simulink model "PitchRateLimiter"  (R2023b)
settings: Solver=FixedStepDiscrete  StartTime=0.0  StopTime=4  FixedStep=Sample_time  RelTol=1e-3
undefined symbols (not defined in the file): q_fallback_command, q_limit_normal, Sample_time
Description:
  | Illustrative 50 Hz pitch-rate command magnitude limiter. Valid normal-mode inputs are clamped inclusively to plus/minus q_limit_normal; invalid or non-normal inputs use q_fallback_command.
settings Model: DataDictionary=FCS_Data.sldd  Creator=Tyler  LastModifiedBy=Tyler
settings CodeAppCC: MaxIdLength=63

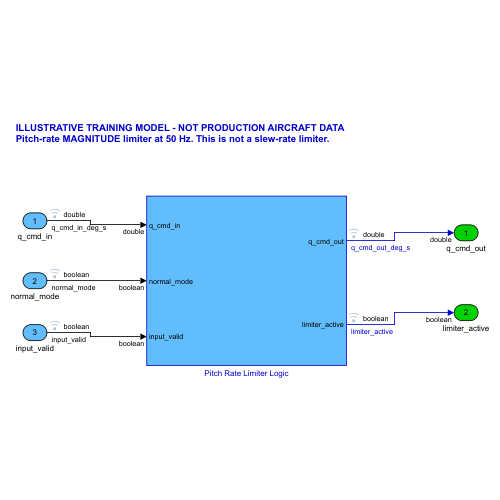
[thumbnail: Simulink's stored preview of the top-level diagram]
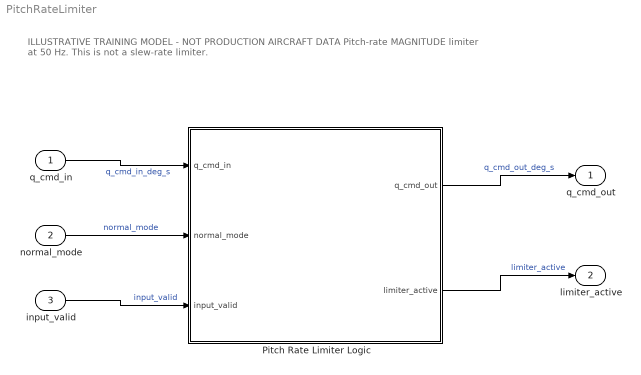
== system PitchRateLimiter ==
  note: ILLUSTRATIVE TRAINING MODEL - NOT PRODUCTION AIRCRAFT DATA
      | Pitch-rate MAGNITUDE limiter at 50 Hz. This is not a slew-rate limiter.
  q_cmd_in : Inport  OutDataTypeStr=double  Unit=deg/s  SampleTime=Sample_time
  normal_mode : Inport  Port=2  OutDataTypeStr=boolean  Unit=1  SampleTime=Sample_time
  input_valid : Inport  Port=3  OutDataTypeStr=boolean  Unit=1  SampleTime=Sample_time
  Pitch Rate Limiter Logic : Subsystem  Description=Inclusive magnitude clamp plus explicit validity/mode fallback. limiter_active is true only while a valid command exceeds a limit.
  q_cmd_out : Outport  OutDataTypeStr=double  Unit=deg/s
  limiter_active : Outport  Port=2  OutDataTypeStr=boolean  Unit=1
  wires:
  q_cmd_in/1 -> Pitch Rate Limiter Logic/1(q_cmd_in)  "q_cmd_in_deg_s"
  normal_mode/1 -> Pitch Rate Limiter Logic/2(normal_mode)  "normal_mode"
  input_valid/1 -> Pitch Rate Limiter Logic/3(input_valid)  "input_valid"
  Pitch Rate Limiter Logic/1(q_cmd_out) -> q_cmd_out/1  "q_cmd_out_deg_s"
  Pitch Rate Limiter Logic/2(limiter_active) -> limiter_active/1  "limiter_active"

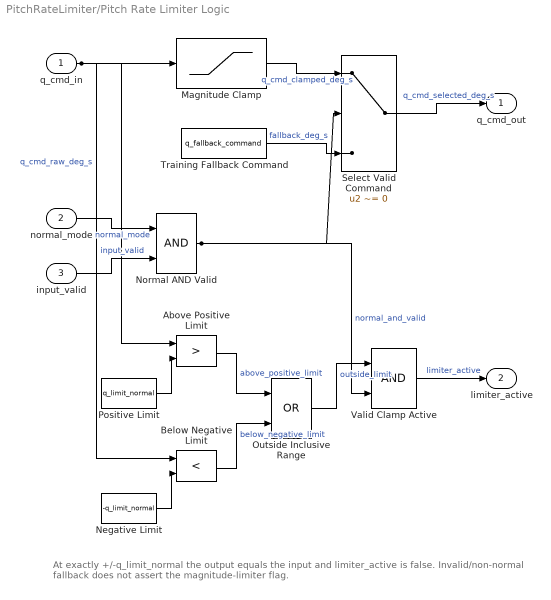
== system PitchRateLimiter/Pitch Rate Limiter Logic ==
  note: At exactly +/-q_limit_normal the output equals the input and limiter_active is false. Invalid/non-normal fallback does not assert the magnitude-limiter flag.
  q_cmd_in : Inport  OutDataTypeStr=double  Unit=deg/s  SampleTime=Sample_time
  normal_mode : Inport  Port=2  OutDataTypeStr=boolean  Unit=1  SampleTime=Sample_time
  input_valid : Inport  Port=3  OutDataTypeStr=boolean  Unit=1  SampleTime=Sample_time
  Above Positive Limit : RelationalOperator  Operator=>  OutDataTypeStr=boolean  RndMeth=Simplest  InputSameDT=off
  Below Negative Limit : RelationalOperator  Operator=<  OutDataTypeStr=boolean  RndMeth=Simplest  InputSameDT=off
  Magnitude Clamp : Saturate  Description=Inclusive command magnitude clamp. This block limits magnitude, not the rate of change of the signal.  UpperLimit=q_limit_normal  LowerLimit=-q_limit_normal
  Negative Limit : Constant  Value=-q_limit_normal  OutDataTypeStr=double  SampleTime=Sample_time
  Normal AND Valid : Logic  AllPortsSameDT=off  OutDataTypeStr=boolean
  Outside Inclusive Range : Logic  Operator=OR  AllPortsSameDT=off  OutDataTypeStr=boolean
  Positive Limit : Constant  Value=q_limit_normal  OutDataTypeStr=double  SampleTime=Sample_time
  Select Valid Command : Switch  Criteria=u2 ~= 0  Threshold=0.5  SaturateOnIntegerOverflow=off  InputSameDT=off
  Training Fallback Command : Constant  Description=Documented training fallback: zero pitch-rate command.  Value=q_fallback_command  OutDataTypeStr=double  SampleTime=Sample_time
  Valid Clamp Active : Logic  AllPortsSameDT=off  OutDataTypeStr=boolean
  q_cmd_out : Outport  OutDataTypeStr=double  Unit=deg/s
  limiter_active : Outport  Port=2  OutDataTypeStr=boolean  Unit=1
  wires:
  normal_mode/1 -> Normal AND Valid/1  "normal_mode"
  input_valid/1 -> Normal AND Valid/2  "input_valid"
  q_cmd_in/1 -> Magnitude Clamp/1, Above Positive Limit/1, Below Negative Limit/1  "q_cmd_raw_deg_s"
  Magnitude Clamp/1 -> Select Valid Command/1  "q_cmd_clamped_deg_s"
  Normal AND Valid/1 -> Select Valid Command/2, Valid Clamp Active/2  "normal_and_valid"
  Training Fallback Command/1 -> Select Valid Command/3  "fallback_deg_s"
  Select Valid Command/1 -> q_cmd_out/1  "q_cmd_selected_deg_s"
  Positive Limit/1 -> Above Positive Limit/2
  Negative Limit/1 -> Below Negative Limit/2
  Above Positive Limit/1 -> Outside Inclusive Range/1  "above_positive_limit"
  Below Negative Limit/1 -> Outside Inclusive Range/2  "below_negative_limit"
  Outside Inclusive Range/1 -> Valid Clamp Active/1  "outside_limit"
  Valid Clamp Active/1 -> limiter_active/1  "limiter_active"
